simulink subsystem "rotorTemp"  (R2023b)
settings: Solver=VariableStepAuto  StartTime=0.0  StopTime=10.0  RelTol=1e-3
libraries: Raptor_lib x4, rotorTemp_lib x4
settings Model: Creator=serga  LastModifiedBy=serga
settings OptimizationCC: ReuseModelBlockBuffer=off

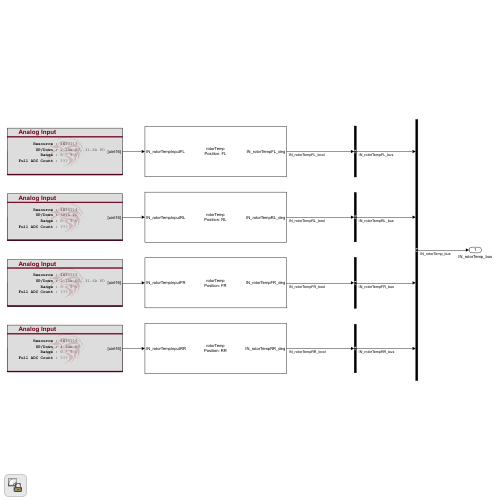
[thumbnail: Simulink's stored preview of the top-level diagram]
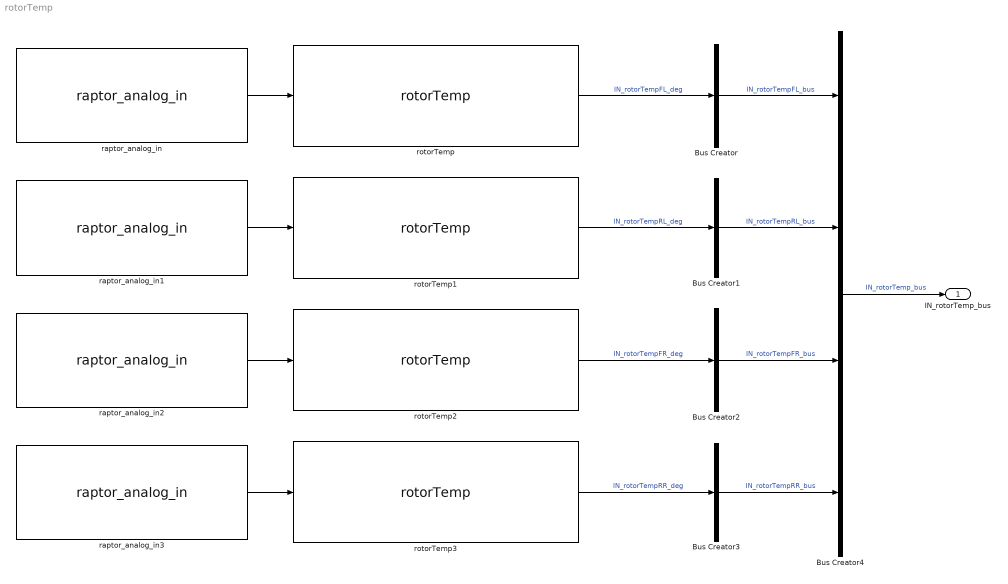
== system rotorTemp ==
  Bus Creator{,1..3} (4 alike) : BusCreator  Inputs=1
  Bus Creator4 : BusCreator  Inputs=4
  raptor_analog_in : Raptor_lib/Input & Output/raptor_analog_in  resourceValues=INPUT2|INPUT3|INPUT4|INPUT5|INPUT6|INPUT7|INPUT8|INPUT9|INPUT10|INPUT11|INPUT12|INPUT13|INPUT14|INPUT15|INPUT16|INPUT17|INPUT18|INPUT19|INPUT20|INPUT21|INPUT22|INPUT23|INPUT24|INPUT25|INPUT26|INPUT27|INPUT28|INPUT29|INPUT30|INPUT31|INPUT32|(None)  resource=INPUT6  rangeValues=0 - 5 V  range=0 - 5 V  filterrateValues=[]  filterrate='RAPTOR MASK DEFAULT'  resolutionValues=[]  resolution=[]  pullUDValues=681k PU  pullUD=681k PU
      settings: SourceProductName=Raptor
  raptor_analog_in1 : Raptor_lib/Input & Output/raptor_analog_in  resourceValues=INPUT2|INPUT3|INPUT4|INPUT5|INPUT6|INPUT7|INPUT8|INPUT9|INPUT10|INPUT11|INPUT12|INPUT13|INPUT14|INPUT15|INPUT16|INPUT17|INPUT18|INPUT19|INPUT20|INPUT21|INPUT22|INPUT23|INPUT24|INPUT25|INPUT26|INPUT27|INPUT28|INPUT29|INPUT30|INPUT31|INPUT32|(None)  resource=INPUT7  rangeValues=0 - 5 V  range=0 - 5 V  filterrateValues=[]  filterrate='RAPTOR MASK DEFAULT'  resolutionValues=[]  resolution=[]  pullUDValues=681k PU  pullUD=681k PU
      settings: SourceProductName=Raptor
  raptor_analog_in2 : Raptor_lib/Input & Output/raptor_analog_in  resourceValues=INPUT2|INPUT3|INPUT4|INPUT5|INPUT6|INPUT7|INPUT8|INPUT9|INPUT10|INPUT11|INPUT12|INPUT13|INPUT14|INPUT15|INPUT16|INPUT17|INPUT18|INPUT19|INPUT20|INPUT21|INPUT22|INPUT23|INPUT24|INPUT25|INPUT26|INPUT27|INPUT28|INPUT29|INPUT30|INPUT31|INPUT32|(None)  resource=INPUT9  rangeValues=0 - 5 V  range=0 - 5 V  filterrateValues=[]  filterrate='RAPTOR MASK DEFAULT'  resolutionValues=[]  resolution=[]  pullUDValues=681k PU  pullUD=681k PU
      settings: SourceProductName=Raptor
  raptor_analog_in3 : Raptor_lib/Input & Output/raptor_analog_in  resourceValues=INPUT2|INPUT3|INPUT4|INPUT5|INPUT6|INPUT7|INPUT8|INPUT9|INPUT10|INPUT11|INPUT12|INPUT13|INPUT14|INPUT15|INPUT16|INPUT17|INPUT18|INPUT19|INPUT20|INPUT21|INPUT22|INPUT23|INPUT24|INPUT25|INPUT26|INPUT27|INPUT28|INPUT29|INPUT30|INPUT31|INPUT32|(None)  resource=INPUT10  rangeValues=0 - 5 V  range=0 - 5 V  filterrateValues=[]  filterrate='RAPTOR MASK DEFAULT'  resolutionValues=[]  resolution=[]  pullUDValues=681k PU  pullUD=681k PU
      settings: SourceProductName=Raptor
  rotorTemp : rotorTemp_lib/rotorTemp  pos='FL'
  rotorTemp1 : rotorTemp_lib/rotorTemp  pos='RL'
  rotorTemp2 : rotorTemp_lib/rotorTemp  pos='FR'
  rotorTemp3 : rotorTemp_lib/rotorTemp  pos='RR'
  IN_rotorTemp_bus : Outport
  wires:
  Bus Creator4/1 -> IN_rotorTemp_bus/1  "IN_rotorTemp_bus"
  Bus Creator3/1 -> Bus Creator4/4  "IN_rotorTempRR_bus"
  Bus Creator2/1 -> Bus Creator4/3  "IN_rotorTempFR_bus"
  Bus Creator1/1 -> Bus Creator4/2  "IN_rotorTempRL_bus"
  Bus Creator/1 -> Bus Creator4/1  "IN_rotorTempFL_bus"
  rotorTemp3/1 -> Bus Creator3/1  "IN_rotorTempRR_deg"
  rotorTemp2/1 -> Bus Creator2/1  "IN_rotorTempFR_deg"
  rotorTemp1/1 -> Bus Creator1/1  "IN_rotorTempRL_deg"
  rotorTemp/1 -> Bus Creator/1  "IN_rotorTempFL_deg"
  raptor_analog_in/1 -> rotorTemp/1
  raptor_analog_in1/1 -> rotorTemp1/1
  raptor_analog_in2/1 -> rotorTemp2/1
  raptor_analog_in3/1 -> rotorTemp3/1
